simulink model "NandiniG_23EEM1S02_hcc"  (R2024b)
settings: Solver=VariableStepAuto  StartTime=0.0  StopTime=1  RelTol=1e-3
libraries: spsIGBTDiodeLib x6, simulink x2, spsPermanentMagnetSynchronousMachineLib x1, spsDCVoltageSourceLib x1, slpidlib x1, spsThreePhaseVIMeasurementLib x1, spspowerguiLib x1
settings Model: Creator=Deepak  LastModifiedBy=INNAGOL2
settings SolverCC: AlgebraicLoopSolver=TrustRegion
settings DebuggingCC: UnconnectedInputMsg=warning  UnconnectedOutputMsg=warning  UnconnectedLineMsg=warning
settings ModelReferenceCC: EnableRefExpFcnMdlSchedulingChecks=on
settings SFSimCC: CustomCodeUndefinedFunction=UseInterfaceOnly
settings RTWCC: GPUComputeCapability=3.5

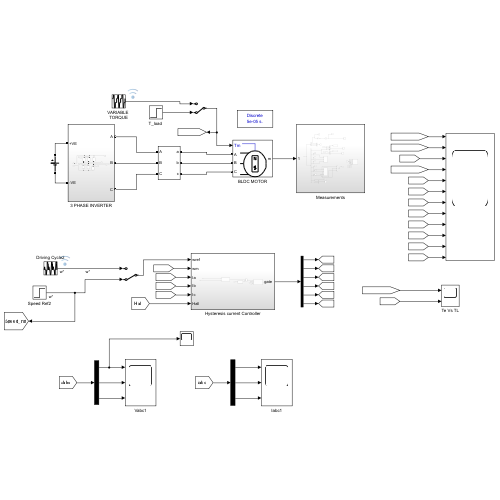
[thumbnail: Simulink's stored preview of the top-level diagram]
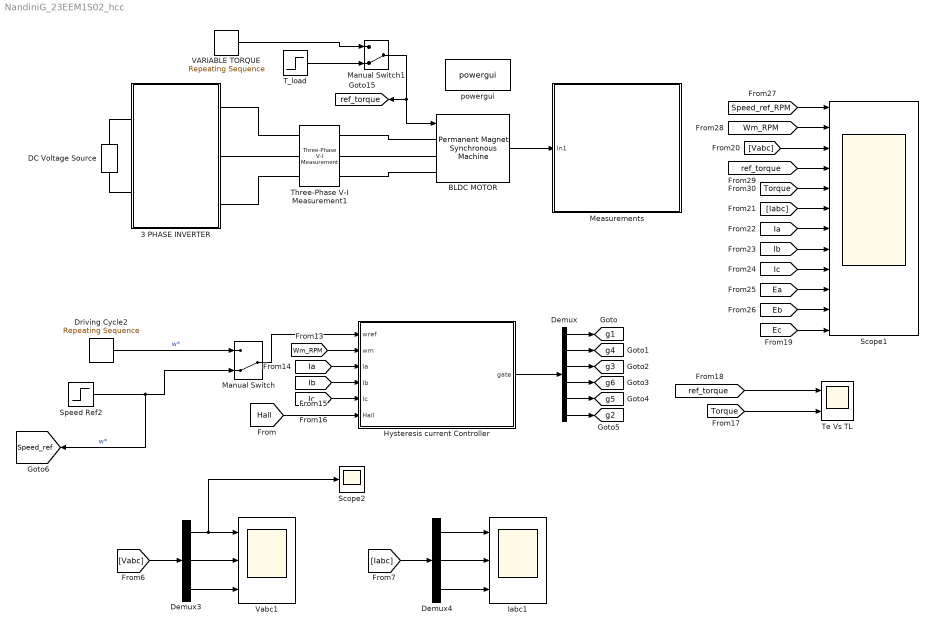
== system NandiniG_23EEM1S02_hcc ==
  3 PHASE INVERTER : Subsystem
  BLDC MOTOR : spsPermanentMagnetSynchronousMachineLib/Permanent Magnet Synchronous Machine  NbPhases=3  FluxDistribution=Trapezoidal  RotorType=Round  MechanicalLoad=Torque Tm  PresetModel=No  ShowDetailedParameters=on  MeasurementBus=off  Resistance=0.7  Inductance=2.7e-3  dqInductances=[8.5e-3,8.5e-3]  La=0.000395  MachineConstant=Flux linkage established by magnets (V.s)  Flux=0.1194  VoltageCst=100.0283  TorqueCst=0.9552  Flat=120  Mechanical=[0.0027 0.0004924 4 0]  PolePairs=4  InitialConditions=[0,0, 0,0]  InitialConditions5ph=[0 0 0 0 0 0]  RefAngle=90 degrees behind phase A axis (modified Park)  IterativeDiscreteModel=Trapezoidal non iterative  TsBlock=-1  TsPowergui=0
  DC Voltage Source : spsDCVoltageSourceLib/DC Voltage Source  Amplitude=160  Measurements=None
  Demux : Demux  Outputs=6
  Demux3 : Demux  Outputs=3
  Demux4 : Demux  Outputs=3
  Driving Cycle2 : simulink/Sources/Repeating Sequence  rep_seq_t=[0 1 2 3 4 5 6 7 8 9 10 11 11.0001 12 13]  rep_seq_y=[0 20 20 0 0 0 -30 -30 0 0 50 50 40 40 0]
  Hysteresis current Controller : Subsystem
  Iabc1 : Scope  NumInputPorts=3
  Manual Switch : ManualSwitch  CurrentSetting=0
  Manual Switch1 : ManualSwitch  CurrentSetting=0
  Measurements : Subsystem
  Scope1 : Scope  NumInputPorts=12
  Scope2 : Scope
  Speed Ref2 : Step  Time=0.1  After=150  SampleTime=0
  "T_load " : Step  Time=0.1  After=5  SampleTime=0
  Te Vs TL : Scope  NumInputPorts=2
  Three-Phase V-I Measurement1 : spsThreePhaseVIMeasurementLib/Three-Phase V-I Measurement  VoltageMeasurement=phase-to-phase  SetLabelV=on  LabelV=Vabc  Vpu=off  VpuLL=off  CurrentMeasurement=yes  SetLabelI=on  LabelI=Iabc  Ipu=off  Pbase=100e6  Vbase=500e3  OutputType=Complex  PhasorSimulation=off  PSBequivalent=0
  VARIABLE TORQUE : simulink/Sources/Repeating Sequence  rep_seq_t=[0 1 2 3 4 5 6 7 8 9 10 11 12 13]  rep_seq_y=[3 3 3 3 5 5 5 -2 -2 -2 1 1 1 1 ]
  Vabc1 : Scope  NumInputPorts=3
  powergui : spspowerguiLib/powergui  Priority=1  SimulationMode=Discrete  SampleTime=5e-05  frequency=60  Iterations=50  frequencyindice=0  Pbase=100e6  ErrMax=1e-4  UnitsV=kV  UnitsW=MW  buscounter=0  FunctionMessages=off  echomessages=off  EnableUseOfTLC=off  CurrentSourceSwitches=off  DisableSnubberDevices=off  DisableRonSwitches=off  DisableVfSwitches=off  DisplayEquations=off  AutomaticDiscreteSolvers=off  SolverType=Tustin/Backward Euler (TBE)  Interpol=off  ExternalGateDelay=off  methode=off  Ts=100  x0status=blocks  SPID=on  SwTol=0  HookPort=off  NonlinearTolerance=0  nMaxIteration=15  ContinueOnMaxIteration=off  RestoreLinks=warning  ResistiveCurrentMeasurement=off  Frange=[0:2:500]  Ylog=off  Xlog=on  ShowGrid=off  save=off  variable=ZData  structure=0  ZoomFFT=off  StartTime=0.0  cycles=1  DisplayStyle=1  fundamental=60  FreqAxis=off  MaxFrequency=1000  frequencyindicesteady=1  RmsSteady=1  display=off
  tag scope: Speed_ref=global, g1=global, g2=global, g3=global, g4=global, g5=global, g6=global, ref_torque=global
  wires:
  Demux/4 -> [g6]
  Demux/3 -> [g3]
  Demux/5 -> [g5]
  Demux/1 -> [g1]
  Demux/6 -> [g2]
  Demux/2 -> [g4]
  [Hall] -> Hysteresis current Controller/6("Hall ")
  [Wm_RPM] -> Hysteresis current Controller/2(wm)
  [Ia] -> Hysteresis current Controller/3(Ia)
  [Ib] -> Hysteresis current Controller/4(Ib)
  [Ic] -> Hysteresis current Controller/5(Ic)
  Hysteresis current Controller/1("gate ") -> Demux/1
  "T_load "/1 -> Manual Switch1/2
  VARIABLE TORQUE/1 -> Manual Switch1/1
  Manual Switch1/1 -> [ref_torque], BLDC MOTOR/1
  Speed Ref2/1 -> [Speed_ref], Manual Switch/2  "w*"
  Manual Switch/1 -> Hysteresis current Controller/1(wref)
  Driving Cycle2/1 -> Manual Switch/1  "w*"
  [ref_torque] -> Te Vs TL/1
  [Torque] -> Te Vs TL/2
  BLDC MOTOR/1 -> Measurements/1(In1)
  [Ea] -> Scope1/10
  [Ic] -> Scope1/9
  [Torque] -> Scope1/5
  [Ec] -> Scope1/12
  [Vabc] -> Scope1/3
  [ref_torque] -> Scope1/4
  [Speed_ref_RPM] -> Scope1/1
  [Ia] -> Scope1/7
  [Iabc] -> Scope1/6
  [Wm_RPM] -> Scope1/2
  [Ib] -> Scope1/8
  [Eb] -> Scope1/11
  Demux3/2 -> Vabc1/2
  Demux4/2 -> Iabc1/2
  [Vabc] -> Demux3/1
  Demux4/3 -> Iabc1/3
  Demux3/1 -> Scope2/1, Vabc1/1
  Demux3/3 -> Vabc1/3
  Demux4/1 -> Iabc1/1
  [Iabc] -> Demux4/1
  connections:
  DC Voltage Source/RConn1 -- 3 PHASE INVERTER/LConn1
  DC Voltage Source/LConn1 -- 3 PHASE INVERTER/LConn2
  3 PHASE INVERTER/RConn1 -- Three-Phase V-I Measurement1/LConn1
  3 PHASE INVERTER/RConn2 -- Three-Phase V-I Measurement1/LConn2
  3 PHASE INVERTER/RConn3 -- Three-Phase V-I Measurement1/LConn3
  Three-Phase V-I Measurement1/RConn1 -- BLDC MOTOR/LConn1
  Three-Phase V-I Measurement1/RConn2 -- BLDC MOTOR/LConn2
  Three-Phase V-I Measurement1/RConn3 -- BLDC MOTOR/LConn3

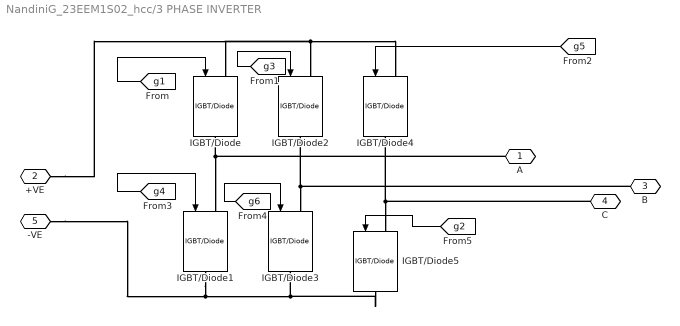
== system NandiniG_23EEM1S02_hcc/3 PHASE INVERTER ==
  IGBT/Diode{,1..5} (6 alike) : spsIGBTDiodeLib/IGBT//Diode  Ron=1e-3  Rs=1e5  Cs=inf  Measurements=off
  A : PMIOPort  Side=Right
  +VE : PMIOPort  Port=2  Side=Left
  B : PMIOPort  Port=3  Side=Right
  C : PMIOPort  Port=4  Side=Right
  -VE : PMIOPort  Port=5  Side=Left
  wires:
  [g1] -> IGBT/Diode/1
  [g3] -> IGBT/Diode2/1
  [g5] -> IGBT/Diode4/1
  [g4] -> IGBT/Diode1/1
  [g6] -> IGBT/Diode3/1
  [g2] -> IGBT/Diode5/1
  connections:
  A/RConn1 -- IGBT/Diode/RConn1 -- IGBT/Diode1/LConn1
  B/RConn1 -- IGBT/Diode2/RConn1 -- IGBT/Diode3/LConn1
  C/RConn1 -- IGBT/Diode4/RConn1 -- IGBT/Diode5/LConn1
  +VE/RConn1 -- IGBT/Diode/LConn1 -- IGBT/Diode2/LConn1 -- IGBT/Diode4/LConn1
  -VE/RConn1 -- IGBT/Diode5/RConn1 -- IGBT/Diode3/RConn1 -- IGBT/Diode1/RConn1

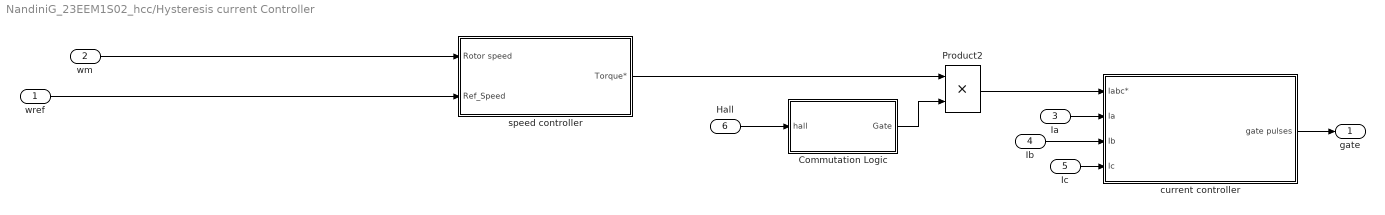
== system NandiniG_23EEM1S02_hcc/Hysteresis current Controller ==
  wref : Inport
  wm : Inport  Port=2
  Ia : Inport  Port=3
  Ib : Inport  Port=4
  Ic : Inport  Port=5
  "Hall " : Inport  Port=6
  Commutation Logic : Subsystem
  Product2 : Product  SaturateOnIntegerOverflow=on  OutDataTypeStr=Inherit: Same as first input
  current controller : Subsystem
  speed controller : Subsystem
  "gate " : Outport  VectorParamsAs1DForOutWhenUnconnected=off
  wires:
  "Hall "/1 -> Commutation Logic/1("hall ")
  Commutation Logic/1(Gate) -> Product2/2
  current controller/1(gate pulses) -> "gate "/1
  Ic/1 -> current controller/4(Ic)
  Ib/1 -> current controller/3(Ib)
  Ia/1 -> current controller/2(Ia)
  Product2/1 -> current controller/1(Iabc*)
  wm/1 -> speed controller/1(Rotor speed)
  speed controller/1(Torque*) -> Product2/1
  wref/1 -> speed controller/2(Ref_Speed)

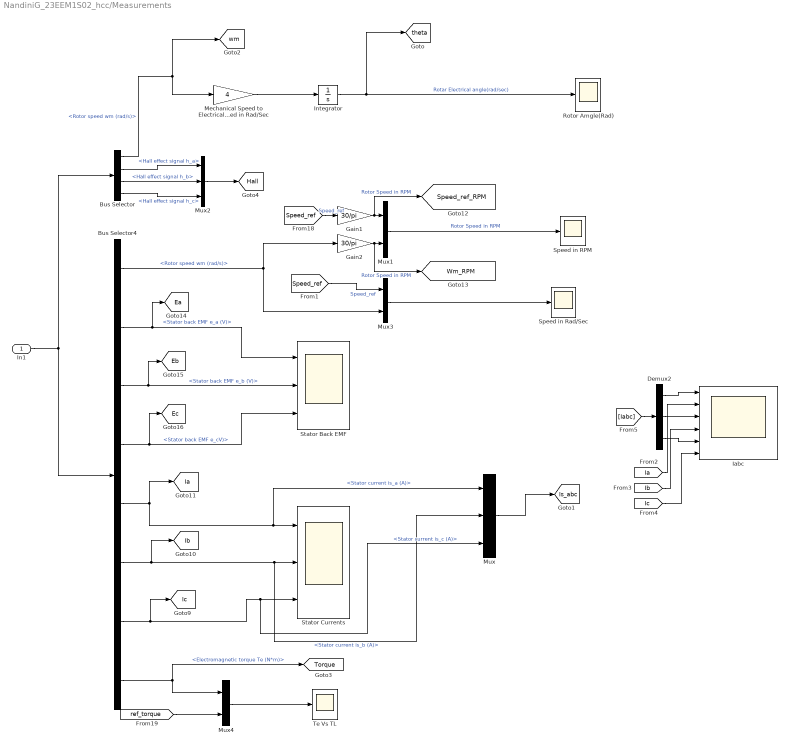
== system NandiniG_23EEM1S02_hcc/Measurements ==
  In1 : Inport
  Bus Selector : BusSelector  OutputSignals=Rotor speed wm (rad/s),Hall effect signal h_a,Hall effect signal h_b,Hall effect signal h_c
  Bus Selector4 : BusSelector  OutputSignals=Rotor speed wm (rad/s),Stator back EMF e_a (V),Stator back EMF e_b (V),Stator back EMF e_cV),Stator current is_a (A),Stator current is_b (A),Stator current is_c (A),Electromagnetic torque Te (N*m)
  Demux2 : Demux  Outputs=3
  Gain1 : Gain  Gain=30/pi
  Gain2 : Gain  Gain=30/pi
  Iabc : Scope  NumInputPorts=6
  Integrator : Integrator  WrapState=on
  Mechanical Speed to Electrical speed in Rad/Sec : Gain  Gain=4
  Mux : Mux  Inputs=3
  Mux1 : Mux  Inputs=2
  Mux2 : Mux  Inputs=3
  Mux3 : Mux  Inputs=2
  Mux4 : Mux  Inputs=2
  Rotor Amgle(Rad) : Scope
  Speed in RPM : Scope
  Speed in Rad/Sec : Scope
  Stator Back EMF : Scope  NumInputPorts=3
  Stator Currents : Scope  NumInputPorts=3
  Te Vs TL : Scope
  tag scope: Ea=global, Eb=global, Ec=global, Hall=global, Ia=global, Ib=global, Ic=global, Is_abc=global, Speed_ref_RPM=global, Torque=global, Wm_RPM=global, theta=global, wm=global
  wires:
  [ref_torque] -> Mux4/2
  Mechanical Speed to Electrical speed in Rad/Sec/1 -> Integrator/1
  Mux4/1 -> Te Vs TL/1
  Bus Selector/1 -> Mechanical Speed to Electrical speed in Rad/Sec/1, [wm]  "<Rotor speed wm (rad/s)>"
  Bus Selector4/3 -> [Eb], Stator Back EMF/2  "<Stator back EMF e_b (V)>"
  Bus Selector4/8 -> [Torque], Mux4/1  "<Electromagnetic torque Te (N*m)>"
  Bus Selector4/5 -> [Ia], Mux/1, Stator Currents/1  "<Stator current is_a (A)>"
  In1/1 -> Bus Selector4/1, Bus Selector/1
  Bus Selector4/4 -> [Ec], Stator Back EMF/3  "<Stator back EMF e_cV)>"
  Gain2/1 -> [Wm_RPM], Mux1/2  "Rotor Speed in RPM"
  Bus Selector4/7 -> [Ic], Mux/3, Stator Currents/3  "<Stator current is_c (A)>"
  Integrator/1 -> [theta], Rotor Amgle(Rad)/1  "Rotar Electrical angle(rad/sec)"
  Bus Selector4/2 -> [Ea], Stator Back EMF/1  "<Stator back EMF e_a (V)>"
  Bus Selector4/1 -> Mux3/2, Gain2/1  "<Rotor speed wm (rad/s)>"
  Gain1/1 -> [Speed_ref_RPM], Mux1/1  "Rotor Speed in RPM"
  Mux3/1 -> Speed in Rad/Sec/1
  Mux1/1 -> Speed in RPM/1  "Rotor Speed in RPM"
  [Speed_ref] -> Gain1/1  "Speed_ref"
  Bus Selector4/6 -> [Ib], Mux/2, Stator Currents/2  "<Stator current is_b (A)>"
  [Speed_ref] -> Mux3/1  "Speed_ref"
  Mux/1 -> [Is_abc]
  Bus Selector/2 -> Mux2/1  "<Hall effect signal h_a>"
  Bus Selector/3 -> Mux2/2  "<Hall effect signal h_b>"
  Bus Selector/4 -> Mux2/3  "<Hall effect signal h_c>"
  Mux2/1 -> [Hall]
  [Ib] -> Iabc/4
  [Ic] -> Iabc/6
  Demux2/2 -> Iabc/3
  Demux2/1 -> Iabc/1
  [Ia] -> Iabc/2
  Demux2/3 -> Iabc/5
  [Iabc] -> Demux2/1

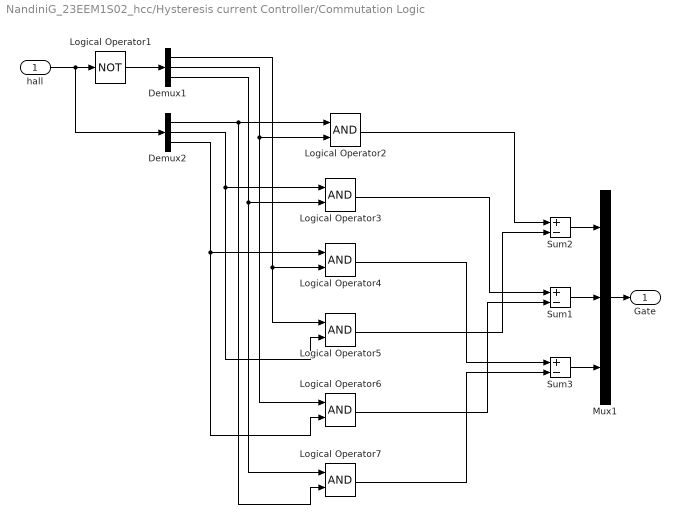
== system NandiniG_23EEM1S02_hcc/Hysteresis current Controller/Commutation Logic ==
  "hall " : Inport
  Demux1 : Demux  Outputs=3
  Demux2 : Demux  Outputs=3
  Logical Operator1 : Logic  Operator=NOT  AllPortsSameDT=off  OutDataTypeStr=boolean
  Logical Operator{2..7} (6 alike) : Logic  AllPortsSameDT=off  OutDataTypeStr=boolean
  Mux1 : Mux  Inputs=3
  Sum1 : Sum  Inputs=+-  OutDataTypeStr=double
  Sum2 : Sum  Inputs=+-  OutDataTypeStr=double
  Sum3 : Sum  Inputs=+-  OutDataTypeStr=double
  Gate : Outport  VectorParamsAs1DForOutWhenUnconnected=off
  wires:
  Demux2/1 -> Logical Operator7/2, Logical Operator2/1
  Demux1/3 -> Logical Operator7/1, Logical Operator3/2
  Demux2/2 -> Logical Operator3/1, Logical Operator5/2
  Sum1/1 -> Mux1/2
  Logical Operator3/1 -> Sum1/1
  "hall "/1 -> Logical Operator1/1, Demux2/1
  Demux1/2 -> Logical Operator6/1, Logical Operator2/2
  Logical Operator2/1 -> Sum2/1
  Logical Operator7/1 -> Sum3/2
  Logical Operator4/1 -> Sum3/1
  Demux1/1 -> Logical Operator4/2, Logical Operator5/1
  Logical Operator6/1 -> Sum1/2
  Logical Operator5/1 -> Sum2/2
  Sum3/1 -> Mux1/3
  Logical Operator1/1 -> Demux1/1
  Mux1/1 -> Gate/1
  Sum2/1 -> Mux1/1
  Demux2/3 -> Logical Operator4/1, Logical Operator6/2

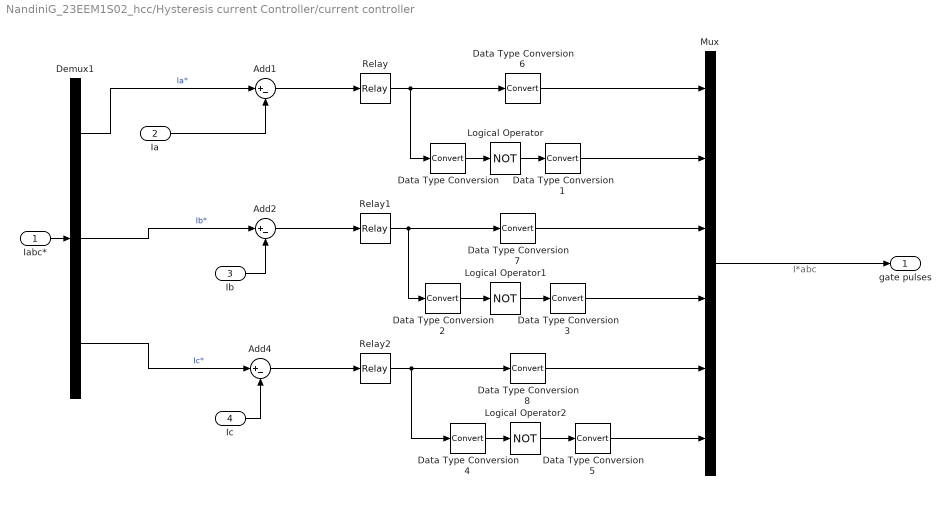
== system NandiniG_23EEM1S02_hcc/Hysteresis current Controller/current controller ==
  note: I*abc
  Iabc* : Inport
  Ia : Inport  Port=2
  Ib : Inport  Port=3
  Ic : Inport  Port=4
  Add1 : Sum  Inputs=|+-
  Add2 : Sum  Inputs=|+-
  Add4 : Sum  Inputs=|+-
  Data Type Conversion{,1..8} (9 alike) : DataTypeConversion
  Demux1 : Demux  Outputs=3
      settings: DisplayOption=none
  Logical Operator : Logic  Operator=NOT  AllPortsSameDT=off  OutDataTypeStr=boolean
  Logical Operator1 : Logic  Operator=NOT  AllPortsSameDT=off  OutDataTypeStr=boolean
  Logical Operator2 : Logic  Operator=NOT  AllPortsSameDT=off  OutDataTypeStr=boolean
  Mux : Mux  Inputs=6
  Relay : Relay  OnSwitchValue=0.1  OffSwitchValue=-0.1
  Relay1 : Relay  OnSwitchValue=0.1  OffSwitchValue=-0.1
  Relay2 : Relay  OnSwitchValue=0.1  OffSwitchValue=-0.1
  gate pulses : Outport  VectorParamsAs1DForOutWhenUnconnected=off
  wires:
  Relay/1 -> Data Type Conversion/1, Data Type Conversion6/1
  Relay1/1 -> Data Type Conversion7/1, Data Type Conversion2/1
  Relay2/1 -> Data Type Conversion8/1, Data Type Conversion4/1
  Ib/1 -> Add2/2
  Mux/1 -> gate pulses/1
  Ic/1 -> Add4/2
  Data Type Conversion/1 -> Logical Operator/1
  Logical Operator/1 -> Data Type Conversion1/1
  Data Type Conversion1/1 -> Mux/2
  Logical Operator1/1 -> Data Type Conversion3/1
  Data Type Conversion3/1 -> Mux/4
  Data Type Conversion2/1 -> Logical Operator1/1
  Data Type Conversion5/1 -> Mux/6
  Logical Operator2/1 -> Data Type Conversion5/1
  Data Type Conversion4/1 -> Logical Operator2/1
  Demux1/2 -> Add2/1  "Ib*"
  Demux1/3 -> Add4/1  "Ic*"
  Iabc*/1 -> Demux1/1
  Ia/1 -> Add1/2
  Demux1/1 -> Add1/1  "Ia*"
  Add1/1 -> Relay/1
  Add2/1 -> Relay1/1
  Data Type Conversion6/1 -> Mux/1
  Data Type Conversion7/1 -> Mux/3
  Data Type Conversion8/1 -> Mux/5
  Add4/1 -> Relay2/1

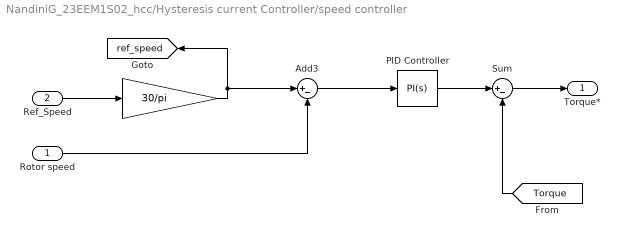
== system NandiniG_23EEM1S02_hcc/Hysteresis current Controller/speed controller ==
  Rotor speed : Inport
  Ref_Speed : Inport  Port=2
  " " : Gain  Gain=30/pi
  Add3 : Sum  Inputs=|+-
  PID Controller : slpidlib/PID Controller  Controller=PI  Form=Parallel  TimeDomain=Continuous-time  UseExternalTs=off  SampleTime=-1  IntegratorMethod=Forward Euler  FilterMethod=Forward Euler  ControllerParametersSource=internal  P=6  I=5  UseKiTs=off  D=0  UseExternalDerivativeSource=off  N=100  UseFilter=on  TunerSelectOption=Transfer Function Based (PID Tuner App)  InitialConditionSource=internal  InitialConditionForIntegrator=0  InitialConditionForFilter=0  DifferentiatorICPrevScaledInput=0  ExternalReset=none  TrackingMode=off  Kt=1  LimitOutput=off  SatLimitsSource=internal  UpperSaturationLimit=10  LowerSaturationLimit=0  LinearizeAsGain=on  AntiWindupMode=none  Kb=1  LimitIntegrator=off  UpperIntegratorSaturationLimit=inf  LowerIntegratorSaturationLimit=-inf  POutMin=[]  POutMax=[]  IOutMin=[]  IOutMax=[]  DOutMin=[]  DOutMax=[]  NOutMin=[]  NOutMax=[]  SumOutMin=[]  SumOutMax=[]  SaturationOutMin=[]  SaturationOutMax=[]  PParamMin=[]  PParamMax=[]  IParamMin=[]  IParamMax=[]  DParamMin=[]  DParamMax=[]  NParamMin=[]  NParamMax=[]  KbParamMin=[]  KbParamMax=[]  KtParamMin=[]  KtParamMax=[]  KbOutMin=[]  KbOutMax=[]  KtOutMin=[]  KtOutMax=[]  IntegratorOutMin=[]  IntegratorOutMax=[]  FilterOutMin=[]  FilterOutMax=[]  SumI1OutMin=[]  SumI1OutMax=[]  SumI2OutMin=[]  SumI2OutMax=[]  SumI3OutMin=[]  SumI3OutMax=[]  SumI4OutMin=[]  SumI4OutMax=[]  SumDOutMin=[]  SumDOutMax=[]  DifferentiatorOutMin=[]  DifferentiatorOutMax=[]  FilterDiffOutCoefMin=[]  FilterDiffOutCoefMax=[]  ReciprocalOutMin=[]  ReciprocalOutMax=[]  SumDenOutMin=[]  SumDenOutMax=[]  SumNumOutMin=[]  SumNumOutMax=[]  DivideOutMin=[]  DivideOutMax=[]  UdiffTsProdOutMin=[]  UdiffTsProdOutMax=[]  NTsProdOutMin=[]  NTsProdOutMax=[]  UintegralTsProdOutMin=[]  UintegralTsProdOutMax=[]  UngainTsProdOutMin=[]  UngainTsProdOutMax=[]  ClampingZeroOutDataTypeStr=Inherit: Inherit via back propagation  ClampingZeroOutMin=[]  ClampingZeroOutMax=[]  FilterDenConstantOutDataTypeStr=Inherit: Inherit via back propagation  FilterDenConstantOutMin=[]  FilterDenConstantOutMax=[]  PCopyOutDataTypeStr=Inherit: Inherit via back propagation  PCopyOutMin=[]  PCopyOutMax=[]  NCopyOutDataTypeStr=Inherit: Inherit via back propagation  NCopyOutMin=[]  NCopyOutMax=[]  IntegratorContinuousStateAttributes=''  IntegratorStateMustResolveToSignalObject=off  IntegratorRTWStateStorageClass=Auto  FilterContinuousStateAttributes=''  FilterStateMustResolveToSignalObject=off  FilterRTWStateStorageClass=Auto  ParallelPVariant=InternalParameters  IdealPVariant=Disabled  IVariant=InternalParameters  DVariant=Disabled  IntegratorVariant=Continuous  SatVariant=Disabled  AWVariant=Passthrough  PCopyVariant=Disabled  TRVariant=Disabled  FdbkBlocksVariant=Forward  IdealPFdbkVariant=Disabled  SatFdbkVariant=Disabled  DerivativeFilterVariant=Disabled  NVariant=Disabled  NCopyVariant=Disabled_SignalSpec  FilterICVariant=Disabled  IntegratorICVariant=InternalICs  ExternalResetVariant=Disabled  TRSumVariant=Passthrough  SumFdbkVariant=Disabled  SumVariant=Sum_PI  TsampFilterVariant=InternalTs  TsampNgainVariant=Passthrough  TsampIntegralVariant=Disabled_SignalSpec  ExternalSaturationOutDataTypeStr=Inherit: Same as second input  DerivativeSourceVariant=Disabled  PreIntVariant=InternalPreInt
  Sum : Sum  Inputs=|+-
  Torque* : Outport  VectorParamsAs1DForOutWhenUnconnected=off
  tag scope: ref_speed=global
  wires:
  Add3/1 -> PID Controller/1
  Rotor speed/1 -> Add3/2
  Ref_Speed/1 -> " "/1
  PID Controller/1 -> Sum/1
  [Torque] -> Sum/2
  Sum/1 -> Torque*/1
  " "/1 -> [ref_speed], Add3/1
